simulink model "digital"  (Simulink 7.5)
settings: Solver=ode45  StartTime=0.0  StopTime=10.0  RelTol=1e-3
libraries: simulink x1
settings Model: Creator=eechris  LastModifiedBy=eechris

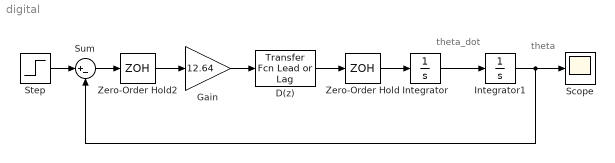
== system digital ==
  note: theta_dot
  note: theta
  D(z) : simulink/Discrete/Transfer Fcn Lead or Lag  SystemSampleTime=-1  PoleZ=0.5488  ZeroZ=0.9051  ICPrevOutput=0.0  ICPrevInput=0.0  DoSatur=off
  Gain : Gain  Gain=12.64  ParameterDataType=fixdt(1, 16)  ParameterScaling=2^0  OutDataType=fixdt(1, 16)  OutScaling=2^0
  Integrator : Integrator
  Integrator1 : Integrator
  Scope : Scope
  Step : Step  SampleTime=0
  Sum : Sum  Inputs=|+-  OutDataType=fixdt(1, 16)  OutScaling=2^0
  Zero-Order Hold : ZeroOrderHold  SampleTime=0.1
  Zero-Order Hold2 : ZeroOrderHold  SampleTime=0.1
  wires:
  Integrator/1 -> Integrator1/1
  Integrator1/1 -> Scope/1, Sum/2
  Zero-Order Hold/1 -> Integrator/1
  ? -> ?
  D(z)/1 -> Zero-Order Hold/1
  Gain/1 -> D(z)/1
  Zero-Order Hold2/1 -> Gain/1
  Sum/1 -> Zero-Order Hold2/1
  Step/1 -> Sum/1
